simulink model "fuzzyLCS"  (R2021b)
settings: Solver=VariableStepAuto  StartTime=0.0  StopTime=10  RelTol=1e-3
undefined symbols (not defined in the file or in its folder): NewD, NewI, NewP
libraries: robotlib x3
settings Model: SimulationMode=accelerator  Creator=lucas  LastModifiedBy=lucas

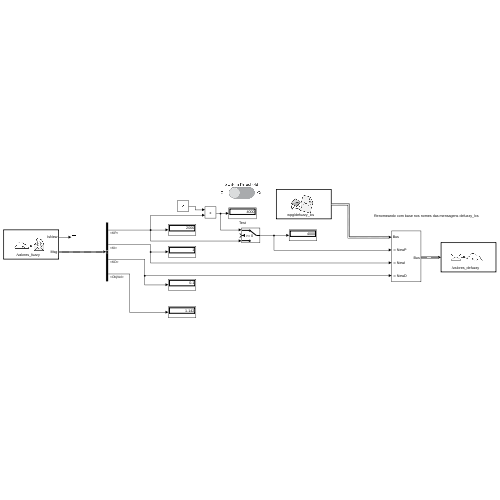
[thumbnail: Simulink's stored preview of the top-level diagram]
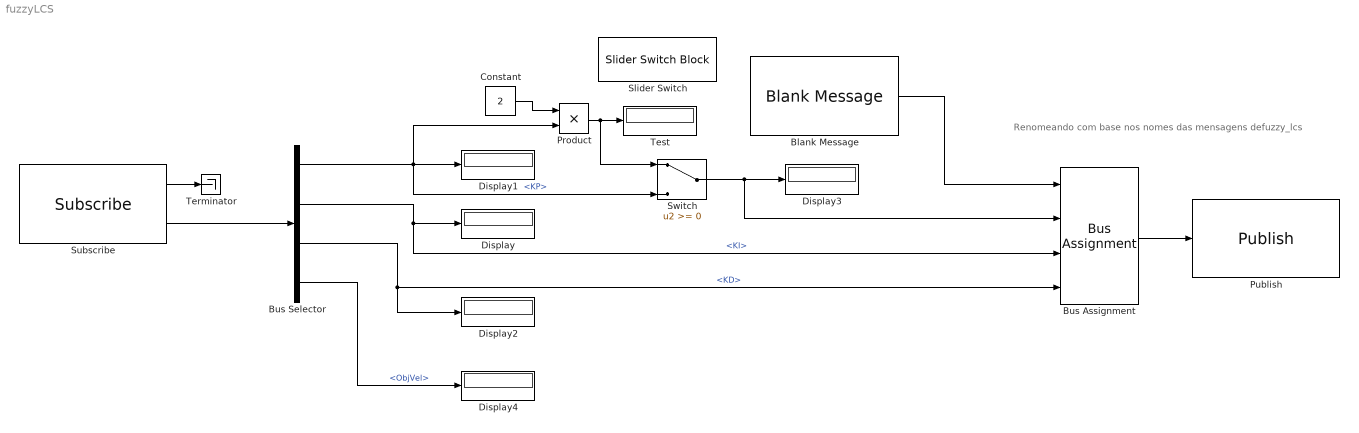
== system fuzzyLCS ==
  note: Renomeando com base nos nomes das mensagens defuzzy_lcs
  Blank Message : robotlib/Blank Message  messageClass=Message  entityType=wpg/defuzzy_lcs  messageType=wpg/defuzzy_lcs  SampleTime=inf  legacyBusStruct=off
  Bus Assignment : BusAssignment  AssignedSignals=NewP,NewI,NewD
  Bus Selector : BusSelector  OutputSignals=KP,KI,KD,ObjVel
  Constant : Constant  Value=2
  Display{,1..4} (5 alike) : Display
      settings: Decimation=2
  Product : Product
  Publish : robotlib/Publish  topicSource=Specify your own  topic=/valores_defuzzy  messageType=wpg/defuzzy_lcs  legacyBusStruct=off  messageQueueLength=1
  Slider Switch : SliderSwitchBlock
      settings: Values={{'Off', 'On'}, [0 1]}
  Subscribe : robotlib/Subscribe  topicSource=Specify your own  topic=/valores_fuzzy  messageType=wpg/fuzzy_lcs  SampleTime=-1  legacyBusStruct=off  messageQueueLength=1
  Switch : Switch
  Terminator : Terminator
  Test : Display
      settings: Decimation=2
  wires:
  Subscribe/2 -> Bus Selector/1
  Subscribe/1 -> Terminator/1
  Bus Selector/1 -> Product/2, Display1/1, Switch/3  "<KP>"
  Bus Selector/2 -> Bus Assignment/3, Display/1  "<KI>"
  Bus Selector/3 -> Display2/1, Bus Assignment/4  "<KD>"
  Constant/1 -> Product/1
  Product/1 -> Switch/1, Test/1
  Switch/1 -> Bus Assignment/2, Display3/1
  Blank Message/1 -> Bus Assignment/1
  Bus Assignment/1 -> Publish/1
  Bus Selector/4 -> Display4/1  "<ObjVel>"
